simulink model "SF051A_SnsrOffsLrng"  (R2013b)
settings: Solver=FixedStepDiscrete  SolverMode=SingleTasking  StartTime=0.0  StopTime=1  FixedStep=0.002  RelTol=1e-3
undefined symbols (not defined in the file): ARCHGLBPRM_10MILLISEC_SEC_F32, ARCHGLBPRM_2MILLISEC_SEC_F32, ARCHGLBPRM_2PI_ULS_F32, ARCHGLBPRM_FLOATZEROTHD_ULS_F32, ARCHGLBPRM_PIOVER180_ULS_F32, CNV100MICROSECTOMILLISEC_MILLISECPERCNT_F32, CNV100MICROSECTOSEC_SECPERCNT_F32, COVRAMTRXNIT_ULS_F32, HWAUTHYTHD_ULS_F32, HWTQLRNGSTSLRND_CNT_U08, HWTQLRNGSTSNEGOFFS_CNT_U08, HWTQLRNGSTSNOTLRND_CNT_U08, HWTQLRNGSTSPOSOFFS_CNT_U08, HWTQLRNGSTSZEROOFFS_CNT_U08, HWTQLRNGTMRHILIM_SEC_F32, IDYMTRX_ULS_F32, IVS10MS_ULSPERSEC_F32, LRNGFILTICON_ULS_F32, NvmGetErrSts1, ONE_ULS_F32, SnsrOffsLrnd, SnsrOffsLrngFctEna, SnsrOffsLrngHwAgLrngDrvgDstThd, SnsrOffsLrngHwAgLrngEna, SnsrOffsLrngHwAgLrngHwVelThd, SnsrOffsLrngHwAgLrngSysTqThd, SnsrOffsLrngHwAgLrngSysTqThdMed, SnsrOffsLrngHwAgLrngSysTqThdTrustd, SnsrOffsLrngHwAgLrngSysTqThdWide, SnsrOffsLrngHwAgLrngTi, SnsrOffsLrngHwAgLrngVehSpdThd, SnsrOffsLrngHwAgLrngYawOffsDbnd, SnsrOffsLrngHwAgLrngYawRateThd, SnsrOffsLrngHwAgOffsLim, SnsrOffsLrngHwTqLrngEna, SnsrOffsLrngHwTqLrngEnaTiThd, SnsrOffsLrngHwTqLrngHwAgDbnd, SnsrOffsLrngHwTqLrngHwAgThd, SnsrOffsLrngHwTqLrngHwTqThd, SnsrOffsLrngHwTqLrngHwTqZeroOffsThd, SnsrOffsLrngHwTqLrngHwVelThd, SnsrOffsLrngHwTqLrngMeasTi, SnsrOffsLrngHwTqLrngMeasTiScar, SnsrOffsLrngHwTqLrngSampleImbThd1, SnsrOffsLrngHwTqLrngSampleImbThd2, SnsrOffsLrngHwTqLrngSampleThd1, SnsrOffsLrngHwTqLrngSampleThd2, SnsrOffsLrngHwTqLrngTiWghtCoeff, SnsrOffsLrngHwTqLrngVehSpdThd, SnsrOffsLrngHwTqOffsLim, SnsrOffsLrngSampleCntForHwTqLrngRst, SnsrOffsLrngTqInpDetnPwrEstimnThd, SnsrOffsLrngTqInpDetnSinGenrAmp, SnsrOffsLrngTqInpDetnSinGenrFrq, SnsrOffsLrngTqInpDetnStg1FilGain, SnsrOffsLrngTqInpDetnStg1WinSize, SnsrOffsLrngTqInpDetnStg2FilGainCen, SnsrOffsLrngTqInpDetnStg2FilGainDwn, SnsrOffsLrngTqInpDetnStg2FilGainUp, SnsrOffsLrngTqInpDetnStg2WinSize ... (+15)
libraries: Fil x34, FixdToFloat x17, FloatToFixd x16, NxtrLim x15, simulink x12, NxtrAbslt x12, NxtrNvM x8, NxtrMin x5, NxtrMath x3
(part 11 of 11)

== system SF051A_SnsrOffsLrng/SnsrOffsLrng/SnsrOffsLrngPer2/Enable_Function/POC/Learn/BiasEstimation_ValidityCheck/HwTqAvrg_Check/Switch Case Action Subsystem4 ==
  SysTqThdTrustd : Inport
  Action Port : ActionPort  ActionType=case
  Gain : Gain  Gain=-1
  Subsystem5 : Subsystem  Description=|  mask(Copyright Information){none=on}
      | Copyright info block.                                               
      |                                                                     
      | Place copyright information at the top of every subsystem in design.
      mask prompts: none "No parameters"
      mask help: Place copyright information at the top of every subsystem in design.
      mask Display:
      | NxtrConf = 'Nexteer Confidential';
      | 
      | sys = bdroot; %handle for the current model ("system")
      | first = get_param(sys,'Created');
      | first = first(end-3:end);  %year is last four digits
      | 
      | last = get_param(sys,'LastModifiedDate');
      | if isempty(last)
      |     last = datestr(now,'yyyy');
      | else
      |     last = last(end-3:end);
      | end
      | 
      | if strcmp(first,last)
      |     fprintf('%s -- Copyright %s Nexteer',NxtrConf,first)
      | else
      |     fprintf('%s -- %s%s- %s Nexteer',NxtrConf,char(169),first,last)
      | end
  UpTh : Outport
  LowTh : Outport  Port=2
  wires:
  Gain/1 -> LowTh/1
  SysTqThdTrustd/1 -> Gain/1, UpTh/1

== system SF051A_SnsrOffsLrng/SnsrOffsLrng/SnsrOffsLrngPer2/Enable_Function/POC/Learn/BiasEstimation_ValidityCheck/HwTqAvrg_Check/Switch Case Action Subsystem5 ==
  SysTqThdWide : Inport
  Action Port : ActionPort  ActionType=default
  Gain : Gain  Gain=-1
  Subsystem5 : Subsystem  Description=|  mask(Copyright Information){none=on}
      | Copyright info block.                                               
      |                                                                     
      | Place copyright information at the top of every subsystem in design.
      mask prompts: none "No parameters"
      mask help: Place copyright information at the top of every subsystem in design.
      mask Display:
      | NxtrConf = 'Nexteer Confidential';
      | 
      | sys = bdroot; %handle for the current model ("system")
      | first = get_param(sys,'Created');
      | first = first(end-3:end);  %year is last four digits
      | 
      | last = get_param(sys,'LastModifiedDate');
      | if isempty(last)
      |     last = datestr(now,'yyyy');
      | else
      |     last = last(end-3:end);
      | end
      | 
      | if strcmp(first,last)
      |     fprintf('%s -- Copyright %s Nexteer',NxtrConf,first)
      | else
      |     fprintf('%s -- %s%s- %s Nexteer',NxtrConf,char(169),first,last)
      | end
  UpTh : Outport
  LowTh : Outport  Port=2
  wires:
  SysTqThdWide/1 -> Gain/1, UpTh/1
  Gain/1 -> LowTh/1

== system SF051A_SnsrOffsLrng/SnsrOffsLrng/SnsrOffsLrngPer2/Enable_Function/POC/Learn/BiasEstimation_ValidityCheck/Keep OR Reset/Limit and Keep Learned Value ==
  HwPosBiasEstRaw : Inport
  Action Port : ActionPort  ActionType=then
  Constant : Constant  RequirementInfo={'linktype_rmi_doors' '0000babd (/E-STEER Core/SubSystem Specifications/Application Functions/SF051A Sensor Offset Learning)' '#SF051A_138' 'true' 'REQ:SF051A_138' '' } %GIDa_21289eda_9e85_4347_9687_653c781a611d  Value=ZERO_ULS_F32  OutDataTypeStr=single
      settings: AttributesFormatString=%<OutDataTypeStr>
  Constant1 : Constant  RequirementInfo={'linktype_rmi_doors' '0000babd (/E-STEER Core/SubSystem Specifications/Application Functions/SF051A Sensor Offset Learning)' '#SF051A_140' 'true' 'REQ:SF051A_140' '' } %GIDa_a6f07fad_f17c_4ace_8365_667990c14b30  Value=SnsrOffsLrngHwAgOffsLim  OutDataTypeStr=single
  FloatToFixd_s16_f32 : FloatToFixd/FloatToFixd_s16_f32  Param1=10
  LimDyn_f32 : NxtrLim/LimDyn_f32  RequirementInfo={'linktype_rmi_doors' '0000babd (/E-STEER Core/SubSystem Specifications/Application Functions/SF051A Sensor Offset Learning)' '#SF051A_140' 'true' 'REQ:SF051A_140' '' } %GIDa_2915a7af_cb2e_4592_b132_f2e0d313b25c
  NVM Ram : DataStoreWrite  RequirementInfo={'linktype_rmi_doors' '0000babd (/E-STEER Core/SubSystem Specifications/Application Functions/SF051A Sensor Offset Learning)' '#SF051A_120' 'true' 'REQ:SF051A_120' '' ; 'linktype_rmi_doors' '0000babd (/E-STEER Core/SubSystem Specifications/Application Functions/SF051A Sensor Offset Learning)' '#SF051A_119' 'true' 'REQ:SF051A_119' '' } %GIDa_c18d5963_4a3f_423e_af1b_c67d16260ba6  DataStoreName=SnsrOffsLrnd  DataStoreElements=SnsrOffsLrnd.HwAgLrndTi#SnsrOffsLrnd.HwAgOffs
  Subsystem5 : Subsystem  Description=|  mask(Copyright Information){none=on}
      | Copyright info block.                                               
      |                                                                     
      | Place copyright information at the top of every subsystem in design.
      mask prompts: none "No parameters"
      mask help: Place copyright information at the top of every subsystem in design.
      mask Display:
      | NxtrConf = 'Nexteer Confidential';
      | 
      | sys = bdroot; %handle for the current model ("system")
      | first = get_param(sys,'Created');
      | first = first(end-3:end);  %year is last four digits
      | 
      | last = get_param(sys,'LastModifiedDate');
      | if isempty(last)
      |     last = datestr(now,'yyyy');
      | else
      |     last = last(end-3:end);
      | end
      | 
      | if strcmp(first,last)
      |     fprintf('%s -- Copyright %s Nexteer',NxtrConf,first)
      | else
      |     fprintf('%s -- %s%s- %s Nexteer',NxtrConf,char(169),first,last)
      | end
  Unary Minus : UnaryMinus  RequirementInfo={'linktype_rmi_doors' '0000babd (/E-STEER Core/SubSystem Specifications/Application Functions/SF051A Sensor Offset Learning)' '#SF051A_140' 'true' 'REQ:SF051A_140' '' } %GIDa_fa7a1a43_c58a_4d89_8cd2_8f38148a6033
  wires:
  Constant/1 -> NVM Ram/1
  LimDyn_f32/1 -> FloatToFixd_s16_f32/1
  Unary Minus/1 -> LimDyn_f32/2
  Constant1/1 -> LimDyn_f32/3, Unary Minus/1
  HwPosBiasEstRaw/1 -> LimDyn_f32/1
  FloatToFixd_s16_f32/1 -> NVM Ram/2

== system SF051A_SnsrOffsLrng/SnsrOffsLrng/SnsrOffsLrngPer2/Enable_Function/POC/Learn/BiasEstimation_ValidityCheck/Keep OR Reset/Reset_HwAgLrng ==
  note: Suggest coding as inline local function: void Reset_HwAg_Learning()
  note: Set HwAg Offlset learning filter back to the last good learned value written to NVM Ram.
      | Set elapsed learning time back to zero.
  note: Reset timer
  note: Reset filters
  Action Port : ActionPort  ActionType=else
  Constant : Constant  RequirementInfo={'linktype_rmi_doors' '0000babd (/E-STEER Core/SubSystem Specifications/Application Functions/SF051A Sensor Offset Learning)' '#SF051A_139' 'true' 'REQ:SF051A_139' '' } %GIDa_4560022c_466c_4507_b52b_9d9e5f5221da  Value=ZERO_ULS_F32  OutDataTypeStr=single
      settings: AttributesFormatString=%<OutDataTypeStr>
  Constant1 : Constant  RequirementInfo={'linktype_rmi_doors' '0000babd (/E-STEER Core/SubSystem Specifications/Application Functions/SF051A Sensor Offset Learning)' '#SF051A_139' 'true' 'REQ:SF051A_139' '' } %GIDa_5e13df5a_3650_4084_aa1a_80989b1f2780  Value=ZERO_ULS_F32  OutDataTypeStr=single
      settings: AttributesFormatString=%<OutDataTypeStr>
  Filter SV : DataStoreWrite  RequirementInfo={'linktype_rmi_doors' '0000babd (/E-STEER Core/SubSystem Specifications/Application Functions/SF051A Sensor Offset Learning)' '#SF051A_139' 'true' 'REQ:SF051A_139' '' } %GIDa_be755dd9_fcb9_4425_99f4_faf64e25047e  DataStoreName=HwAgLrngFil1  DataStoreElements=HwAgLrngFil1.FilSt
  Filter SV1 : DataStoreWrite  RequirementInfo={'linktype_rmi_doors' '0000babd (/E-STEER Core/SubSystem Specifications/Application Functions/SF051A Sensor Offset Learning)' '#SF051A_139' 'true' 'REQ:SF051A_139' '' } %GIDa_db09f921_4b2f_4c4a_a571_f8085cef7377  DataStoreName=HwAgLrngFil2  DataStoreElements=HwAgLrngFil2.FilSt
  Filter SV2 : DataStoreWrite  RequirementInfo={'linktype_rmi_doors' '0000babd (/E-STEER Core/SubSystem Specifications/Application Functions/SF051A Sensor Offset Learning)' '#SF051A_139' 'true' 'REQ:SF051A_139' '' } %GIDa_eca337dd_6526_4b71_a1b3_c946e62c85db  DataStoreName=HwAgLrngSysTqFil1  DataStoreElements=HwAgLrngSysTqFil1.FilSt
  Filter SV3 : DataStoreWrite  RequirementInfo={'linktype_rmi_doors' '0000babd (/E-STEER Core/SubSystem Specifications/Application Functions/SF051A Sensor Offset Learning)' '#SF051A_139' 'true' 'REQ:SF051A_139' '' } %GIDa_b7490b1d_2567_4876_95c7_4a522d04e094  DataStoreName=HwAgLrngSysTqFil2  DataStoreElements=HwAgLrngSysTqFil2.FilSt
  FixdToFloat_f32_s16 : FixdToFloat/FixdToFloat_f32_s16  RequirementInfo={'linktype_rmi_doors' '0000babd (/E-STEER Core/SubSystem Specifications/Application Functions/SF051A Sensor Offset Learning)' '#SF051A_139' 'true' 'REQ:SF051A_139' '' } %GIDa_07f227f4_e48d_450e_941a_caccc55d408c  Param1=10
  FloatToFixd_s16_f1 : FloatToFixd/FloatToFixd_s16_f32  RequirementInfo={'linktype_rmi_doors' '0000babd (/E-STEER Core/SubSystem Specifications/Application Functions/SF051A Sensor Offset Learning)' '#SF051A_139' 'true' 'REQ:SF051A_139' '' } %GIDa_9f4cd521_c682_414e_8f7b_f4d8bb8d08d8  Param1=4
  FloatToFixd_s16_f32 : FloatToFixd/FloatToFixd_s16_f32  RequirementInfo={'linktype_rmi_doors' '0000babd (/E-STEER Core/SubSystem Specifications/Application Functions/SF051A Sensor Offset Learning)' '#SF051A_139' 'true' 'REQ:SF051A_139' '' } %GIDa_eb1dd361_8662_488a_ae55_706cff78fefd  Param1=5
  NVMRam_Read : DataStoreRead  RequirementInfo={'linktype_rmi_doors' '0000babd (/E-STEER Core/SubSystem Specifications/Application Functions/SF051A Sensor Offset Learning)' '#SF051A_139' 'true' 'REQ:SF051A_139' '' } %GIDa_177ac313_4fc5_4d7a_9c86_b1caf788b8ab  DataStoreName=SnsrOffsLrnd  DataStoreElements=SnsrOffsLrnd.YawRateOffs
  Read NVM Ram : DataStoreRead  RequirementInfo={'linktype_rmi_doors' '0000babd (/E-STEER Core/SubSystem Specifications/Application Functions/SF051A Sensor Offset Learning)' '#SF051A_139' 'true' 'REQ:SF051A_139' '' } %GIDa_cc646748_aa1c_414f_b217_a4a1e7ec684c  DataStoreName=SnsrOffsLrnd  DataStoreElements=SnsrOffsLrnd.HwAgOffs
  Subsystem5 : Subsystem  Description=|  mask(Copyright Information){none=on}
      | Copyright info block.                                               
      |                                                                     
      | Place copyright information at the top of every subsystem in design.
      mask prompts: none "No parameters"
      mask help: Place copyright information at the top of every subsystem in design.
      mask Display:
      | NxtrConf = 'Nexteer Confidential';
      | 
      | sys = bdroot; %handle for the current model ("system")
      | first = get_param(sys,'Created');
      | first = first(end-3:end);  %year is last four digits
      | 
      | last = get_param(sys,'LastModifiedDate');
      | if isempty(last)
      |     last = datestr(now,'yyyy');
      | else
      |     last = last(end-3:end);
      | end
      | 
      | if strcmp(first,last)
      |     fprintf('%s -- Copyright %s Nexteer',NxtrConf,first)
      | else
      |     fprintf('%s -- %s%s- %s Nexteer',NxtrConf,char(169),first,last)
      | end
  Update Reference : DataStoreWrite  RequirementInfo={'linktype_rmi_doors' '0000babd (/E-STEER Core/SubSystem Specifications/Application Functions/SF051A Sensor Offset Learning)' '#SF051A_139' 'true' 'REQ:SF051A_139' '' } %GIDa_1dfc11a1_5f56_44a1_bae8_84f200f7324d  DataStoreName=SnsrOffsLrnd  DataStoreElements=SnsrOffsLrnd.HwAgLrngYawOffsRef
  Write NVM Ram : DataStoreWrite  RequirementInfo={'linktype_rmi_doors' '0000babd (/E-STEER Core/SubSystem Specifications/Application Functions/SF051A Sensor Offset Learning)' '#SF051A_139' 'true' 'REQ:SF051A_139' '' } %GIDa_39324f37_a93b_47b6_9df3_ec328393f6b7  DataStoreName=SnsrOffsLrnd  DataStoreElements=SnsrOffsLrnd.HwAgLrndTi
  Write NVM Ram1 : DataStoreWrite  RequirementInfo={'linktype_rmi_doors' '0000babd (/E-STEER Core/SubSystem Specifications/Application Functions/SF051A Sensor Offset Learning)' '#SF051A_139' 'true' 'REQ:SF051A_139' '' } %GIDa_e39abcc7_e566_46cb_a681_dee0ec267987  DataStoreName=SnsrOffsLrnd  DataStoreElements=SnsrOffsLrnd.HwAgLrngHwAgFilSt#SnsrOffsLrnd.HwAgLrngSysTqFilSt
  wires:
  Constant/1 -> Write NVM Ram/1
  NVMRam_Read/1 -> Update Reference/1
  Read NVM Ram/1 -> FixdToFloat_f32_s16/1
  Constant1/1 -> Filter SV3/1, Filter SV2/1, FloatToFixd_s16_f32/1
  FixdToFloat_f32_s16/1 -> Filter SV/1, FloatToFixd_s16_f1/1, Filter SV1/1
  FloatToFixd_s16_f1/1 -> Write NVM Ram1/1
  FloatToFixd_s16_f32/1 -> Write NVM Ram1/2

== system SF051A_SnsrOffsLrng/SnsrOffsLrng/SnsrOffsLrngPer2/Enable_Function/POC/Learn/BiasEstimation_ValidityCheck/Keep OR Reset/Subsystem5 ==

== system SF051A_SnsrOffsLrng/SnsrOffsLrng/SnsrOffsLrngPer2/Enable_Function/POC/Learn/BiasEstimation_ValidityCheck/Time_Check/Subsystem5 ==

== system SF051A_SnsrOffsLrng/SnsrOffsLrng/SnsrOffsLrngPer1/EnableLearning/Perform_TqInpDetn/Enable_PreProcessing/Preprocessing/General_Goertzel/Goertzel_Part1_1/Subsystem5 ==

== system SF051A_SnsrOffsLrng/SnsrOffsLrng/SnsrOffsLrngPer1/EnableLearning/Perform_TqInpDetn/Enable_PreProcessing/Preprocessing/General_Goertzel/Goertzel_Part1_2/Subsystem5 ==

== system SF051A_SnsrOffsLrng/SnsrOffsLrng/SnsrOffsLrngPer1/EnableLearning/Perform_TqInpDetn/Enable_PreProcessing/Preprocessing/General_Goertzel/Goertzel_Part1_3/Subsystem5 ==

== system SF051A_SnsrOffsLrng/SnsrOffsLrng/SnsrOffsLrngPer1/EnableLearning/Perform_TqInpDetn/Enable_PreProcessing/Preprocessing/NewOut_ResetCntr/Goertzel_Part2_1/Subsystem5 ==

== system SF051A_SnsrOffsLrng/SnsrOffsLrng/SnsrOffsLrngPer1/EnableLearning/Perform_TqInpDetn/Enable_PreProcessing/Preprocessing/NewOut_ResetCntr/Goertzel_Part2_2/Subsystem5 ==

== system SF051A_SnsrOffsLrng/SnsrOffsLrng/SnsrOffsLrngPer1/EnableLearning/Perform_TqInpDetn/Enable_PreProcessing/Preprocessing/NewOut_ResetCntr/Goertzel_Part2_3/Subsystem5 ==

== system SF051A_SnsrOffsLrng/SnsrOffsLrng/SnsrOffsLrngPer1/EnableLearning/Perform_TqInpDetn/Enable_PreProcessing/Preprocessing/Sliding_Goertzel_ver001/SinGen/Angle_Wrapper ==
  note: To avoid, potential overflow problems, phase angle is being wrapped every 2*pi (equivalent of 360 deg) interval.
  AgIn : Inport
  Constant : Constant  Value=ARCHGLBPRM_2PI_ULS_F32
  EndIf : Merge
  If : If  IfExpression=u1
  Pass_Thru : Subsystem  TreatAsAtomicUnit=on
  Relational Operator : RelationalOperator  OutDataTypeStr=boolean
  Subsystem5 : Subsystem  Description=|  mask(Copyright Information){none=on}
      | Copyright info block.                                               
      |                                                                     
      | Place copyright information at the top of every subsystem in design.
      mask prompts: none "No parameters"
      mask help: Place copyright information at the top of every subsystem in design.
      mask Display:
      | NxtrConf = 'Nexteer Confidential';
      | 
      | sys = bdroot; %handle for the current model ("system")
      | first = get_param(sys,'Created');
      | first = first(end-3:end);  %year is last four digits
      | 
      | last = get_param(sys,'LastModifiedDate');
      | if isempty(last)
      |     last = datestr(now,'yyyy');
      | else
      |     last = last(end-3:end);
      | end
      | 
      | if strcmp(first,last)
      |     fprintf('%s -- Copyright %s Nexteer',NxtrConf,first)
      | else
      |     fprintf('%s -- %s%s- %s Nexteer',NxtrConf,char(169),first,last)
      | end
  Wrap_Angle : Subsystem  TreatAsAtomicUnit=on
  AgOut : Outport
  wires:
  If/1 -> Wrap_Angle/Action
  Wrap_Angle/1(AgOut) -> EndIf/1
  Pass_Thru/1(AgOut) -> EndIf/2
  AgIn/1 -> [AgIn], Pass_Thru/1(AgIn), Relational Operator/1
  If/2 -> Pass_Thru/Action
  EndIf/1 -> AgOut/1
  [AgIn] -> Wrap_Angle/1(AgIn)
  Constant/1 -> Relational Operator/2
  Relational Operator/1 -> If/1

== system SF051A_SnsrOffsLrng/SnsrOffsLrng/SnsrOffsLrngPer1/EnableLearning/Perform_TqInpDetn/Enable_PreProcessing/Preprocessing/Sliding_Goertzel_ver001/SinGen/Convert_To_Radians ==
  note: Output of this block is the increase in the phase angle per time step.
  Freq : Inport
  Constant : Constant  Value=ARCHGLBPRM_2PI_ULS_F32
  Product : Product  RndMeth=Zero
  Product1 : Product  RndMeth=Zero
  Subsystem5 : Subsystem  Description=|  mask(Copyright Information){none=on}
      | Copyright info block.                                               
      |                                                                     
      | Place copyright information at the top of every subsystem in design.
      mask prompts: none "No parameters"
      mask help: Place copyright information at the top of every subsystem in design.
      mask Display:
      | NxtrConf = 'Nexteer Confidential';
      | 
      | sys = bdroot; %handle for the current model ("system")
      | first = get_param(sys,'Created');
      | first = first(end-3:end);  %year is last four digits
      | 
      | last = get_param(sys,'LastModifiedDate');
      | if isempty(last)
      |     last = datestr(now,'yyyy');
      | else
      |     last = last(end-3:end);
      | end
      | 
      | if strcmp(first,last)
      |     fprintf('%s -- Copyright %s Nexteer',NxtrConf,first)
      | else
      |     fprintf('%s -- %s%s- %s Nexteer',NxtrConf,char(169),first,last)
      | end
  time_step : Constant  Value=ARCHGLBPRM_2MILLISEC_SEC_F32
  PhaAgStep : Outport
  wires:
  Constant/1 -> Product/2
  Product/1 -> Product1/1
  time_step/1 -> Product1/2
  Freq/1 -> Product/1
  Product1/1 -> PhaAgStep/1  "PhaAgStep"

== system SF051A_SnsrOffsLrng/SnsrOffsLrng/SnsrOffsLrngPer1/EnableLearning/Perform_TqInpDetn/Enable_PreProcessing/Preprocessing/Sliding_Goertzel_ver001/SinGen/Subsystem5 ==

== system SF051A_SnsrOffsLrng/SnsrOffsLrng/SnsrOffsLrngPer1/EnableLearning/Perform_TqInpDetn/Enable_PreProcessing/Preprocessing/Sliding_Goertzel_ver001/SlidingGoertzel/Calculate_Magnitude ==
  x_n : Inport
  Constant : Constant  Value=SnsrOffsLrngTqInpDetnStg1FilGain
  Constant1 : Constant  Value=SnsrOffsLrngTqInpDetnStg1FilGain
  Data Store Read : DataStoreRead  Priority=1  DataStoreName=TqInpDetnStg1FilSt1
      settings: AttributesFormatString=priority: %<Priority>
  Data Store Read1 : DataStoreRead  Priority=1  DataStoreName=TqInpDetnStg1FilSt2
  Data Store Read2 : DataStoreRead  Priority=2  DataStoreName=TqInpDetnStg1FilSt1
      settings: AttributesFormatString=priority: %<Priority>
  Data Store Write : DataStoreWrite  Priority=3  DataStoreName=TqInpDetnStg1FilSt1
      settings: AttributesFormatString=priority: %<Priority>
  Data Store Write1 : DataStoreWrite  Priority=2  DataStoreName=TqInpDetnStg1FilSt2
      settings: AttributesFormatString=priority: %<Priority>
  Goertzel_Part1 : Subsystem  TreatAsAtomicUnit=on
      settings: RTWSystemCode=Inline
  Goertzel_Part2 : Subsystem  TreatAsAtomicUnit=on
      settings: RTWSystemCode=Inline
  Subsystem5 : Subsystem  Description=|  mask(Copyright Information){none=on}
      | Copyright info block.                                               
      |                                                                     
      | Place copyright information at the top of every subsystem in design.
      mask prompts: none "No parameters"
      mask help: Place copyright information at the top of every subsystem in design.
      mask Display:
      | NxtrConf = 'Nexteer Confidential';
      | 
      | sys = bdroot; %handle for the current model ("system")
      | first = get_param(sys,'Created');
      | first = first(end-3:end);  %year is last four digits
      | 
      | last = get_param(sys,'LastModifiedDate');
      | if isempty(last)
      |     last = datestr(now,'yyyy');
      | else
      |     last = last(end-3:end);
      | end
      | 
      | if strcmp(first,last)
      |     fprintf('%s -- Copyright %s Nexteer',NxtrConf,first)
      | else
      |     fprintf('%s -- %s%s- %s Nexteer',NxtrConf,char(169),first,last)
      | end
  MgnSq : Outport  OutDataTypeStr=single
  wires:
  x_n/1 -> Goertzel_Part1/1(X0)
  Goertzel_Part1/1(S0) -> Data Store Write/1, Goertzel_Part2/1(S0)  "FiltSt0"
  Data Store Read1/1 -> Goertzel_Part1/3(S2)
  Constant/1 -> Goertzel_Part1/2(FiltGain)
  Constant1/1 -> Goertzel_Part2/3(FiltGain)
  Goertzel_Part2/1(MgnSq) -> MgnSq/1
  Data Store Read2/1 -> Data Store Write1/1
  Data Store Read/1 -> Goertzel_Part2/2(S1), Goertzel_Part1/4(S1)  "FiltSt1"

== system SF051A_SnsrOffsLrng/SnsrOffsLrng/SnsrOffsLrngPer1/EnableLearning/Perform_TqInpDetn/Enable_PreProcessing/Preprocessing/Sliding_Goertzel_ver001/SlidingGoertzel/Sliding_Input ==
  note: Replace oldest with newest.
  note: Current value - oldest value.
  note: To simulate a sliding window, this routine manipulates an array of previous values whose useful length is defined by calibration
      | (total length is defined by the cal's EngMax property).  It treats the useful portion of the array as circular, indexing by one and
      | then wrapping back to zero.
      |
      | When entering this block, the index contains the oldest data in the buffer.  It is used and then replaced by the current value for later use.
      | When leaving this block,  the index contains the newest data in the buffer.
  note: Increment or wrap index for next loop
  HwTq : Inport
  Add : Sum
  Assignment : Assignment  IndexMode=Zero-based  IndexOptions=Index vector (port)  Indices=1  OutputSizes=1
  Constant : Constant  Value=SnsrOffsLrngTqInpDetnStg1WinSize
  Constant1 : Constant  OutDataTypeStr=uint8
      settings: AttributesFormatString=%<OutDataTypeStr>
  Data Store Read : DataStoreRead  DataStoreName=TqInpDetnStg1Buf
  Data Store Read1 : DataStoreRead  DataStoreName=TqInpDetnStg1Idx
  Data Store Read2 : DataStoreRead  DataStoreName=TqInpDetnStg1Buf
  Data Store Read3 : DataStoreRead  DataStoreName=TqInpDetnStg1Idx
  Data Store Write : DataStoreWrite  DataStoreName=TqInpDetnStg1Buf
  Data Store Write1 : DataStoreWrite  DataStoreName=TqInpDetnStg1Idx
  If : If  IfExpression=u1
  Increment_Idx : Subsystem  TreatAsAtomicUnit=on
  Merge : Merge
  Relational Operator : RelationalOperator  OutDataTypeStr=boolean
  Selector : Selector  IndexMode=Zero-based  InputPortWidth=72  IndexOptions=Index vector (port)  Indices=[1 3]  OutputSizes=1
      settings: AttributesFormatString=|
      | Input Width:  %<InputPortWidth>
      | Simulink won't allow a DataDict.Constant.
  Subsystem5 : Subsystem  Description=|  mask(Copyright Information){none=on}
      | Copyright info block.                                               
      |                                                                     
      | Place copyright information at the top of every subsystem in design.
      mask prompts: none "No parameters"
      mask help: Place copyright information at the top of every subsystem in design.
      mask Display:
      | NxtrConf = 'Nexteer Confidential';
      | 
      | sys = bdroot; %handle for the current model ("system")
      | first = get_param(sys,'Created');
      | first = first(end-3:end);  %year is last four digits
      | 
      | last = get_param(sys,'LastModifiedDate');
      | if isempty(last)
      |     last = datestr(now,'yyyy');
      | else
      |     last = last(end-3:end);
      | end
      | 
      | if strcmp(first,last)
      |     fprintf('%s -- Copyright %s Nexteer',NxtrConf,first)
      | else
      |     fprintf('%s -- %s%s- %s Nexteer',NxtrConf,char(169),first,last)
      | end
  Subtract : Sum  Inputs=+-
  Wrap_Idx : Subsystem  TreatAsAtomicUnit=on
  x_n : Outport
  wires:
  Selector/1 -> Subtract/2
  Subtract/1 -> x_n/1
  HwTq/1 -> Subtract/1, Assignment/2
  Constant1/1 -> Add/2
  Data Store Read1/1 -> Selector/2
  If/1 -> Wrap_Idx/Action
  Add/1 -> Increment_Idx/1(TqInpDetnStg1IdxIn), Relational Operator/1
  Data Store Read/1 -> Selector/1
  Data Store Read2/1 -> Assignment/1
  Data Store Read3/1 -> Assignment/3, Add/1
  Assignment/1 -> Data Store Write/1
  If/2 -> Increment_Idx/Action
  Merge/1 -> Data Store Write1/1
  Increment_Idx/1(TqInpDetnStg1IdxOut) -> Merge/2
  Wrap_Idx/1(TqInpDetnStg1Idx) -> Merge/1
  Constant/1 -> Relational Operator/2
  Relational Operator/1 -> If/1

== system SF051A_SnsrOffsLrng/SnsrOffsLrng/SnsrOffsLrngPer1/EnableLearning/Perform_TqInpDetn/Enable_PreProcessing/Preprocessing/Sliding_Goertzel_ver001/SlidingGoertzel/Subsystem5 ==

== system SF051A_SnsrOffsLrng/SnsrOffsLrng/SnsrOffsLrngPer2/Enable_Function/POC/Learn/BiasEstimation_ValidityCheck/HwTqAvrg_Check/Switch Case Action Subsystem1/Subsystem5 ==

== system SF051A_SnsrOffsLrng/SnsrOffsLrng/SnsrOffsLrngPer2/Enable_Function/POC/Learn/BiasEstimation_ValidityCheck/HwTqAvrg_Check/Switch Case Action Subsystem2/Subsystem5 ==

== system SF051A_SnsrOffsLrng/SnsrOffsLrng/SnsrOffsLrngPer2/Enable_Function/POC/Learn/BiasEstimation_ValidityCheck/HwTqAvrg_Check/Switch Case Action Subsystem3/Subsystem5 ==

== system SF051A_SnsrOffsLrng/SnsrOffsLrng/SnsrOffsLrngPer2/Enable_Function/POC/Learn/BiasEstimation_ValidityCheck/HwTqAvrg_Check/Switch Case Action Subsystem4/Subsystem5 ==

== system SF051A_SnsrOffsLrng/SnsrOffsLrng/SnsrOffsLrngPer2/Enable_Function/POC/Learn/BiasEstimation_ValidityCheck/HwTqAvrg_Check/Switch Case Action Subsystem5/Subsystem5 ==

== system SF051A_SnsrOffsLrng/SnsrOffsLrng/SnsrOffsLrngPer2/Enable_Function/POC/Learn/BiasEstimation_ValidityCheck/Keep OR Reset/Limit and Keep Learned Value/Subsystem5 ==

== system SF051A_SnsrOffsLrng/SnsrOffsLrng/SnsrOffsLrngPer2/Enable_Function/POC/Learn/BiasEstimation_ValidityCheck/Keep OR Reset/Reset_HwAgLrng/Subsystem5 ==

== system SF051A_SnsrOffsLrng/SnsrOffsLrng/SnsrOffsLrngPer1/EnableLearning/Perform_TqInpDetn/Enable_PreProcessing/Preprocessing/Sliding_Goertzel_ver001/SinGen/Angle_Wrapper/Pass_Thru ==
  AgIn : Inport
  Action Port : ActionPort  ActionType=else
  Subsystem5 : Subsystem  Description=|  mask(Copyright Information){none=on}
      | Copyright info block.                                               
      |                                                                     
      | Place copyright information at the top of every subsystem in design.
      mask prompts: none "No parameters"
      mask help: Place copyright information at the top of every subsystem in design.
      mask Display:
      | NxtrConf = 'Nexteer Confidential';
      | 
      | sys = bdroot; %handle for the current model ("system")
      | first = get_param(sys,'Created');
      | first = first(end-3:end);  %year is last four digits
      | 
      | last = get_param(sys,'LastModifiedDate');
      | if isempty(last)
      |     last = datestr(now,'yyyy');
      | else
      |     last = last(end-3:end);
      | end
      | 
      | if strcmp(first,last)
      |     fprintf('%s -- Copyright %s Nexteer',NxtrConf,first)
      | else
      |     fprintf('%s -- %s%s- %s Nexteer',NxtrConf,char(169),first,last)
      | end
  AgOut : Outport
  wires:
  AgIn/1 -> AgOut/1

== system SF051A_SnsrOffsLrng/SnsrOffsLrng/SnsrOffsLrngPer1/EnableLearning/Perform_TqInpDetn/Enable_PreProcessing/Preprocessing/Sliding_Goertzel_ver001/SinGen/Angle_Wrapper/Subsystem5 ==

== system SF051A_SnsrOffsLrng/SnsrOffsLrng/SnsrOffsLrngPer1/EnableLearning/Perform_TqInpDetn/Enable_PreProcessing/Preprocessing/Sliding_Goertzel_ver001/SinGen/Angle_Wrapper/Wrap_Angle ==
  AgIn : Inport
  Action Port : ActionPort  ActionType=then
  Constant : Constant  Value=ARCHGLBPRM_2PI_ULS_F32
  Subsystem5 : Subsystem  Description=|  mask(Copyright Information){none=on}
      | Copyright info block.                                               
      |                                                                     
      | Place copyright information at the top of every subsystem in design.
      mask prompts: none "No parameters"
      mask help: Place copyright information at the top of every subsystem in design.
      mask Display:
      | NxtrConf = 'Nexteer Confidential';
      | 
      | sys = bdroot; %handle for the current model ("system")
      | first = get_param(sys,'Created');
      | first = first(end-3:end);  %year is last four digits
      | 
      | last = get_param(sys,'LastModifiedDate');
      | if isempty(last)
      |     last = datestr(now,'yyyy');
      | else
      |     last = last(end-3:end);
      | end
      | 
      | if strcmp(first,last)
      |     fprintf('%s -- Copyright %s Nexteer',NxtrConf,first)
      | else
      |     fprintf('%s -- %s%s- %s Nexteer',NxtrConf,char(169),first,last)
      | end
  Subtract : Sum  Inputs=+-
  AgOut : Outport
  wires:
  AgIn/1 -> Subtract/1
  Constant/1 -> Subtract/2
  Subtract/1 -> AgOut/1

== system SF051A_SnsrOffsLrng/SnsrOffsLrng/SnsrOffsLrngPer1/EnableLearning/Perform_TqInpDetn/Enable_PreProcessing/Preprocessing/Sliding_Goertzel_ver001/SinGen/Convert_To_Radians/Subsystem5 ==

== system SF051A_SnsrOffsLrng/SnsrOffsLrng/SnsrOffsLrngPer1/EnableLearning/Perform_TqInpDetn/Enable_PreProcessing/Preprocessing/Sliding_Goertzel_ver001/SlidingGoertzel/Calculate_Magnitude/Goertzel_Part1 ==
  note: s(n-2)
  note: Suggested Coding:  This can be an inline local function.  Simulink limitations prevent modeling it that way, so this block
      | is replicated multiple times throughout the component model.
  X0 : Inport
  FiltGain : Inport  Port=2
  S2 : Inport  Port=3
  S1 : Inport  Port=4
  " Product1" : Product  Inputs=**
  Add1 : Sum  Inputs=++-
  Subsystem5 : Subsystem  Description=|  mask(Copyright Information){none=on}
      | Copyright info block.                                               
      |                                                                     
      | Place copyright information at the top of every subsystem in design.
      mask prompts: none "No parameters"
      mask help: Place copyright information at the top of every subsystem in design.
      mask Display:
      | NxtrConf = 'Nexteer Confidential';
      | 
      | sys = bdroot; %handle for the current model ("system")
      | first = get_param(sys,'Created');
      | first = first(end-3:end);  %year is last four digits
      | 
      | last = get_param(sys,'LastModifiedDate');
      | if isempty(last)
      |     last = datestr(now,'yyyy');
      | else
      |     last = last(end-3:end);
      | end
      | 
      | if strcmp(first,last)
      |     fprintf('%s -- Copyright %s Nexteer',NxtrConf,first)
      | else
      |     fprintf('%s -- %s%s- %s Nexteer',NxtrConf,char(169),first,last)
      | end
  S0 : Outport
  wires:
  Add1/1 -> S0/1
  " Product1"/1 -> Add1/2
  S2/1 -> Add1/3
  FiltGain/1 -> " Product1"/1
  X0/1 -> Add1/1
  S1/1 -> " Product1"/2

== system SF051A_SnsrOffsLrng/SnsrOffsLrng/SnsrOffsLrngPer1/EnableLearning/Perform_TqInpDetn/Enable_PreProcessing/Preprocessing/Sliding_Goertzel_ver001/SlidingGoertzel/Calculate_Magnitude/Goertzel_Part2 ==
  note: abs(y(n))^2
  note: Suggested Coding:  This can be an inline local function.  Simulink limitations prevent modeling it that way, so this block
      | is replicated multiple times throughout the component model.
  note: s^2(n)
  note: s^2(n-1)
  note: s(n-1)
  note: In the academic definition of the goertzel algorithm this block would have a complex calculation.
      | Since we are only interested in the magnitude, the following is an implementation that only need real calculations.
  S0 : Inport
  S1 : Inport  Port=2
  FiltGain : Inport  Port=3
  " Product5" : Product  Inputs=**
  Product2 : Product  Inputs=**
  Product3 : Product  Inputs=**
  Product4 : Product  Inputs=**
  Subsystem5 : Subsystem  Description=|  mask(Copyright Information){none=on}
      | Copyright info block.                                               
      |                                                                     
      | Place copyright information at the top of every subsystem in design.
      mask prompts: none "No parameters"
      mask help: Place copyright information at the top of every subsystem in design.
      mask Display:
      | NxtrConf = 'Nexteer Confidential';
      | 
      | sys = bdroot; %handle for the current model ("system")
      | first = get_param(sys,'Created');
      | first = first(end-3:end);  %year is last four digits
      | 
      | last = get_param(sys,'LastModifiedDate');
      | if isempty(last)
      |     last = datestr(now,'yyyy');
      | else
      |     last = last(end-3:end);
      | end
      | 
      | if strcmp(first,last)
      |     fprintf('%s -- Copyright %s Nexteer',NxtrConf,first)
      | else
      |     fprintf('%s -- %s%s- %s Nexteer',NxtrConf,char(169),first,last)
      | end
  add : Sum  Inputs=++-
  MgnSq : Outport
  wires:
  FiltGain/1 -> " Product5"/2
  add/1 -> MgnSq/1
  Product2/1 -> add/1  "FiltSt0Sq"
  Product3/1 -> add/2  "FiltSt1Sq"
  Product4/1 -> " Product5"/1
  " Product5"/1 -> add/3  "FiltSt0St1"
  S1/1 -> Product3/2, Product3/1, Product4/2
  S0/1 -> Product4/1, Product2/2, Product2/1

== system SF051A_SnsrOffsLrng/SnsrOffsLrng/SnsrOffsLrngPer1/EnableLearning/Perform_TqInpDetn/Enable_PreProcessing/Preprocessing/Sliding_Goertzel_ver001/SlidingGoertzel/Calculate_Magnitude/Subsystem5 ==

== system SF051A_SnsrOffsLrng/SnsrOffsLrng/SnsrOffsLrngPer1/EnableLearning/Perform_TqInpDetn/Enable_PreProcessing/Preprocessing/Sliding_Goertzel_ver001/SlidingGoertzel/Sliding_Input/Increment_Idx ==
  TqInpDetnStg1IdxIn : Inport
  Action Port : ActionPort  ActionType=else
  Subsystem5 : Subsystem  Description=|  mask(Copyright Information){none=on}
      | Copyright info block.                                               
      |                                                                     
      | Place copyright information at the top of every subsystem in design.
      mask prompts: none "No parameters"
      mask help: Place copyright information at the top of every subsystem in design.
      mask Display:
      | NxtrConf = 'Nexteer Confidential';
      | 
      | sys = bdroot; %handle for the current model ("system")
      | first = get_param(sys,'Created');
      | first = first(end-3:end);  %year is last four digits
      | 
      | last = get_param(sys,'LastModifiedDate');
      | if isempty(last)
      |     last = datestr(now,'yyyy');
      | else
      |     last = last(end-3:end);
      | end
      | 
      | if strcmp(first,last)
      |     fprintf('%s -- Copyright %s Nexteer',NxtrConf,first)
      | else
      |     fprintf('%s -- %s%s- %s Nexteer',NxtrConf,char(169),first,last)
      | end
  TqInpDetnStg1IdxOut : Outport
  wires:
  TqInpDetnStg1IdxIn/1 -> TqInpDetnStg1IdxOut/1

== system SF051A_SnsrOffsLrng/SnsrOffsLrng/SnsrOffsLrngPer1/EnableLearning/Perform_TqInpDetn/Enable_PreProcessing/Preprocessing/Sliding_Goertzel_ver001/SlidingGoertzel/Sliding_Input/Subsystem5 ==

== system SF051A_SnsrOffsLrng/SnsrOffsLrng/SnsrOffsLrngPer1/EnableLearning/Perform_TqInpDetn/Enable_PreProcessing/Preprocessing/Sliding_Goertzel_ver001/SlidingGoertzel/Sliding_Input/Wrap_Idx ==
  Action Port : ActionPort  ActionType=then
  Constant : Constant  Value=0  OutDataTypeStr=uint8
      settings: AttributesFormatString=%<OutDataTypeStr>
  Subsystem5 : Subsystem  Description=|  mask(Copyright Information){none=on}
      | Copyright info block.                                               
      |                                                                     
      | Place copyright information at the top of every subsystem in design.
      mask prompts: none "No parameters"
      mask help: Place copyright information at the top of every subsystem in design.
      mask Display:
      | NxtrConf = 'Nexteer Confidential';
      | 
      | sys = bdroot; %handle for the current model ("system")
      | first = get_param(sys,'Created');
      | first = first(end-3:end);  %year is last four digits
      | 
      | last = get_param(sys,'LastModifiedDate');
      | if isempty(last)
      |     last = datestr(now,'yyyy');
      | else
      |     last = last(end-3:end);
      | end
      | 
      | if strcmp(first,last)
      |     fprintf('%s -- Copyright %s Nexteer',NxtrConf,first)
      | else
      |     fprintf('%s -- %s%s- %s Nexteer',NxtrConf,char(169),first,last)
      | end
  TqInpDetnStg1Idx : Outport
  wires:
  Constant/1 -> TqInpDetnStg1Idx/1

== system SF051A_SnsrOffsLrng/SnsrOffsLrng/SnsrOffsLrngPer1/EnableLearning/Perform_TqInpDetn/Enable_PreProcessing/Preprocessing/Sliding_Goertzel_ver001/SinGen/Angle_Wrapper/Pass_Thru/Subsystem5 ==

== system SF051A_SnsrOffsLrng/SnsrOffsLrng/SnsrOffsLrngPer1/EnableLearning/Perform_TqInpDetn/Enable_PreProcessing/Preprocessing/Sliding_Goertzel_ver001/SinGen/Angle_Wrapper/Wrap_Angle/Subsystem5 ==

== system SF051A_SnsrOffsLrng/SnsrOffsLrng/SnsrOffsLrngPer1/EnableLearning/Perform_TqInpDetn/Enable_PreProcessing/Preprocessing/Sliding_Goertzel_ver001/SlidingGoertzel/Calculate_Magnitude/Goertzel_Part1/Subsystem5 ==

== system SF051A_SnsrOffsLrng/SnsrOffsLrng/SnsrOffsLrngPer1/EnableLearning/Perform_TqInpDetn/Enable_PreProcessing/Preprocessing/Sliding_Goertzel_ver001/SlidingGoertzel/Calculate_Magnitude/Goertzel_Part2/Subsystem5 ==

== system SF051A_SnsrOffsLrng/SnsrOffsLrng/SnsrOffsLrngPer1/EnableLearning/Perform_TqInpDetn/Enable_PreProcessing/Preprocessing/Sliding_Goertzel_ver001/SlidingGoertzel/Sliding_Input/Increment_Idx/Subsystem5 ==

== system SF051A_SnsrOffsLrng/SnsrOffsLrng/SnsrOffsLrngPer1/EnableLearning/Perform_TqInpDetn/Enable_PreProcessing/Preprocessing/Sliding_Goertzel_ver001/SlidingGoertzel/Sliding_Input/Wrap_Idx/Subsystem5 ==
